simulink model "mhe"  (R2012b)
settings: Solver=ode45  StartTime=0.0  StopTime=20  RelTol=1e-3
settings Model: Creator=John  LastModifiedBy=John

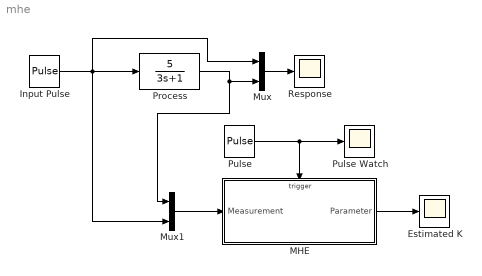
== system mhe ==
  Estimated K : Scope
      settings: SaveName=ScopeData2
  Input Pulse : DiscretePulseGenerator  PulseType=Time based  Amplitude=10  Period=5  PulseWidth=50
  MHE : Subsystem  TreatAsAtomicUnit=on
  Mux : Mux  Inputs=2
  Mux1 : Mux  Inputs=2
  Process : TransferFcn  Numerator=[5]  Denominator=[3 1]
  Pulse : DiscretePulseGenerator  PulseType=Time based  Period=0.2  PulseWidth=5
  Pulse Watch : Scope
  Response : Scope
  wires:
  Input Pulse/1 -> Mux1/2, Mux/1, Process/1
  Mux/1 -> Response/1
  Process/1 -> Mux1/1, Mux/2
  Pulse/1 -> Pulse Watch/1, MHE/Trigger
  MHE/1(Parameter) -> Estimated K/1
  Mux1/1 -> MHE/1(Measurement)

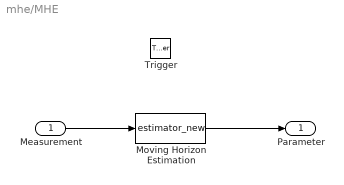
== system mhe/MHE ==
  Measurement : Inport  PortDimensions=2
  Trigger : TriggerPort
  Moving Horizon Estimation : MATLABFcn  MATLABFcn=estimator_new
  Parameter : Outport
  wires:
  Measurement/1 -> Moving Horizon Estimation/1
  Moving Horizon Estimation/1 -> Parameter/1
